simulink model "observador_orden_reducido"  (R2023b)
settings: Solver=VariableStepAuto  StartTime=0.0  StopTime=10.0  RelTol=1e-3
values from neighbouring files (symbols this model uses):
  J_eq = J_m + J_l/(r^2)    (= 1.97847222222e-05)    [constantes.m]    (also in test_polos_PID.m = J_m + J_l/(r^2))
  Ke_theta = 6.4e3    (= 6400)    [constantes.m]
  Ke_w = 1.024e7    (= 10240000)    [constantes.m]
settings Model: Creator=rodri  LastModifiedBy=Nahuel

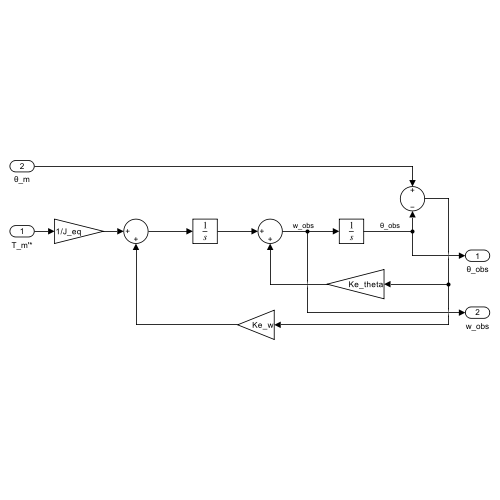
[thumbnail: Simulink's stored preview of the top-level diagram]
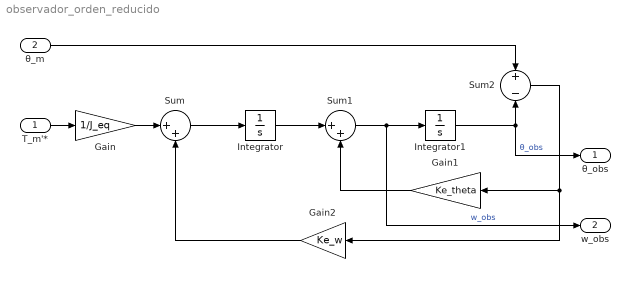
== system observador_orden_reducido ==
  T_m'* : Inport
  θ_m : Inport  Port=2
  Gain : Gain  Gain=1/J_eq
  Gain1 : Gain  Gain=Ke_theta
  Gain2 : Gain  Gain=Ke_w
  Integrator : Integrator
  Integrator1 : Integrator
  Sum : Sum  Inputs=|++
  Sum1 : Sum  Inputs=|++
  Sum2 : Sum  Inputs=+-
  θ_obs : Outport
  w_obs : Outport  Port=2
  wires:
  T_m'*/1 -> Gain/1
  Gain/1 -> Sum/1
  Sum/1 -> Integrator/1
  Integrator/1 -> Sum1/1
  Sum1/1 -> w_obs/1, Integrator1/1  "w_obs"
  Integrator1/1 -> θ_obs/1, Sum2/2  "θ_obs"
  θ_m/1 -> Sum2/1
  Sum2/1 -> Gain2/1, Gain1/1
  Gain1/1 -> Sum1/2
  Gain2/1 -> Sum/2
